simulink model "SEWSYS_Combined"  (Simulink 6.0)
settings: Solver=FixedStepDiscrete  SolverMode=SingleTasking  StartTime=0  StopTime=Q  FixedStep=1  RelTol=1e-3
values from neighbouring files (symbols this model uses):
  andpt = 1/3    (= 0.333333333333)    [constants_trafik.m]
  andt = 0.1    [constants_trafik.m]
  baseflow = str2num(get(HH, 'String'))    [inputs.m]
  CSO_limit = in_CSO_limit    [Prep.m]
  delayinit = [zeros(1,nr_ex_H2O)]    [constants_trafik.m]
  fast = 0.7    [constants_trafik.m]
  fkmday = in_fkmday    [areas.m]
  init_init = 4*3600    (= 14400)    [areas.m]
  init_time = 5    [areas.m]
  nhv = in_nhv/100    [areas.m]
  nr_ex_H2O = totnr-1    (= 20)    [Prep.m]
  numberOfPersons = in_numberOfPersons    [Prep.m]
  othera = in_otherarea    [areas.m]
  othermax = drydepmax*othera    [constants_trafik.m]
  redu = 0.8    [areas.m]
  roada = in_roads    [areas.m]
  roadaccmax = dryper*24*sph*fast*(p_tyrewear+p_roadwear+p_exhaust+p_breakwear+p_drydep+p_corrZn+p_oildischarge+p_catalyst)    [constants_trafik.m]
  roadkm = 67e9    (= 67000000000)    [constants_trafik.m]
  roadrunpart = 1    [constants_trafik.m]
  roadwear = 130000    [constants_trafik.m]
  roadZna = in_part_roadZna/100*roada    [areas.m]
  roofa = in_roofs    [areas.m]
  RoofCua = in_part_roofCua/100*roofa/cos(15*pi/180)    [areas.m]
  roofmax = (Znroofmax*RoofZna+Curoofmax*RoofCua)*roofrunpart+drydepmax*roofa    [constants_trafik.m]
  roofrunpart = 0.7    [constants_trafik.m]
  RoofZna = in_part_roofZna/100*roofa/cos(15*pi/180)    [areas.m]
  sec_per_ts = in_sec_per_ts    [Prep.m]
  sph = 3600/sec_per_ts    [Prep.m]
  tota = in_tota    [areas.m]
  totnr = 21    [Prep.m]
  tyrewear = 9000    [constants_trafik.m]
  wetdep = [sum(s_wetdep(:,i))]*tota*trans1    [polldistr_gr.m]
  yearly_rain = 1    [Callback_simulate.m]    (also in SEWSYS_fig.m)
undefined symbols (not defined in the file or in its folder): BDT, BODofVS, brakep, catalystp, CSO_choice, Curoofp, DiscIntNeverNeededParam, Drainage, drydep, exhp, Faeces, Industry, K, oilp, ProcSS_bio, ProcSS_chem, ProcSS_presed, ProcSS_sand, ProcSS_screen, roadp, sani, spBiooxidBod, spBiored, spCcontent, spChemFe, spChemicalPart, spCODBOD, spDenSS, spHeavym, spHjust, spN2ONpurEmitted, spNemitted, spNitrif, spNpur, spOcontent, spPBound, spPout, spPout1, spVSofSS, SSred_bio, SSred_chem, SSred_presed, SSred_sand, SSred_screen, SStoWater, stormw, tyrep, Urine, VSofSS_sand, VSofSS_screen, Znroofp
(part 1 of 2)
settings Model: LastModifiedBy=v94ahlst  ExtModeTrigMode=oneshot  ExtModeArmWhenConnect=off
settings DataIOCC: LimitDataPoints=off  SignalLoggingName=sigsOut
settings OptimizationCC: BlockReduction=off  BooleanDataType=off
settings DebuggingCC: SolverPrmCheckMsg=none
settings HardwareCC: TargetUnknown=on
settings GRTTargetCC: ModelReferenceCompliant=off  MatFileLogging=off

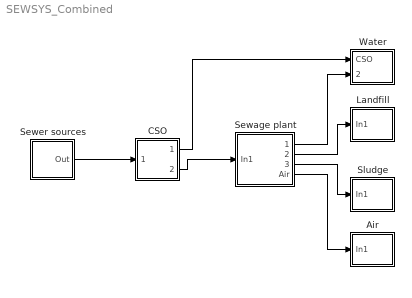
== system SEWSYS_Combined ==
  Air : Subsystem
  CSO : Subsystem
  Landfill : Subsystem
  Sewage plant : Subsystem
  Sewer sources : Subsystem
  Sludge : Subsystem
  Water : Subsystem
  wires:
  Sewage plant/2(Landfill) -> Landfill/1(In1)
  Sewage plant/3(Sludge) -> Sludge/1(In1)
  Sewage plant/1(" Wastewater") -> Water/2(WWTP)
  Sewage plant/4(Air) -> Air/1(In1)
  Sewer sources/1(Out) -> CSO/1(In1)
  CSO/1(Out1) -> Water/1(CSO)
  CSO/2("Out2 ") -> Sewage plant/1(In1)

== system SEWSYS_Combined/Air ==
  In1 : Inport  Port=1  LatchInput=off
  To Workspace : ToWorkspace  VariableName=outAir  SampleTime=-1  SaveFormat=Array
  wires:
  In1/1 -> To Workspace/1

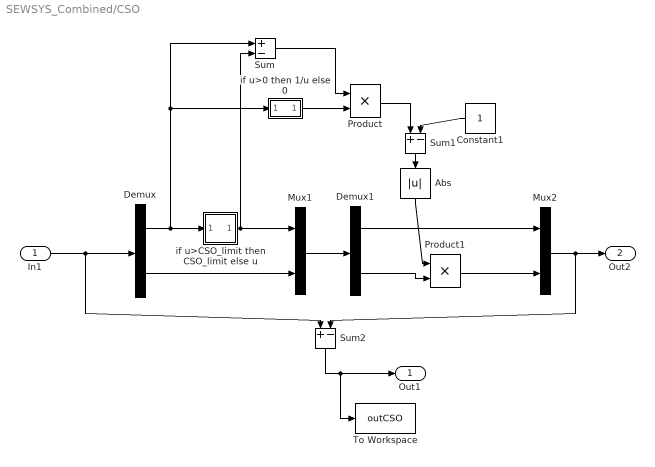
== system SEWSYS_Combined/CSO ==
  In1 : Inport  Port=1  LatchInput=off
  Abs : Abs  Orientation=down  SaturateOnIntegerOverflow=on
  Constant1 : Constant  Orientation=left
  Demux : Demux  Outputs=[1 -1]
  Demux1 : Demux  Outputs=[1 -1]
  Mux1 : Mux  Inputs=2
  Mux2 : Mux  Inputs=2
  Product : Product  SaturateOnIntegerOverflow=on  InputSameDT=on
  Product1 : Product  SaturateOnIntegerOverflow=on  InputSameDT=on
  Sum : Sum  Inputs=+-  SaturateOnIntegerOverflow=on  InputSameDT=on
  Sum1 : Sum  Orientation=down  Inputs=+-  SaturateOnIntegerOverflow=on  InputSameDT=on
  Sum2 : Sum  Orientation=down  Inputs=+-  SaturateOnIntegerOverflow=on  InputSameDT=on
  To Workspace : ToWorkspace  VariableName=outCSO  SampleTime=-1  SaveFormat=Array
  if u>0 then 1/u else 0 : Subsystem
      mask Display: disp('1/u')
  if u>CSO_limit then CSO_limit else u : Subsystem
      mask Display: disp('CSO')
  Out1 : Outport
  "Out2 " : Outport  Port=2
  wires:
  Demux/2 -> Mux1/2
  Mux1/1 -> Demux1/1
  Demux1/1 -> Mux2/1
  Demux1/2 -> Product1/2
  Product1/1 -> Mux2/2
  if u>CSO_limit then CSO_limit else u/1(out_1) -> Sum/2, Mux1/1
  Constant1/1 -> Sum1/2
  Demux/1 -> if u>CSO_limit then CSO_limit else u/1(in_1), Sum/1, if u>0 then 1/u else 0/1(in_1)
  Sum1/1 -> Abs/1
  if u>0 then 1/u else 0/1(out_1) -> Product/2
  Sum2/1 -> Out1/1, To Workspace/1
  In1/1 -> Demux/1, Sum2/1
  Mux2/1 -> "Out2 "/1, Sum2/2
  Product/1 -> Sum1/1
  Abs/1 -> Product1/1
  Sum/1 -> Product/1

== system SEWSYS_Combined/Landfill ==
  In1 : Inport  Port=1  LatchInput=off
  To Workspace : ToWorkspace  VariableName=outLandfill  SampleTime=-1  SaveFormat=Array
  wires:
  In1/1 -> To Workspace/1

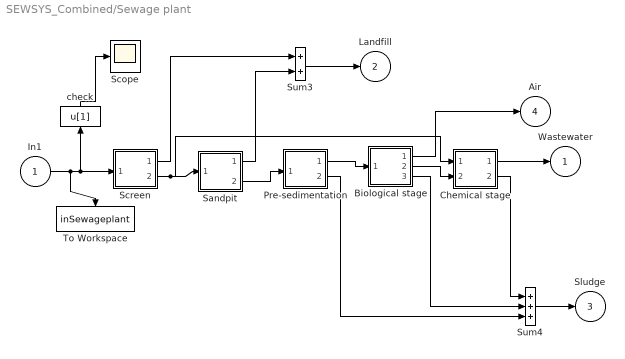
== system SEWSYS_Combined/Sewage plant ==
  In1 : Inport  Port=1  LatchInput=off
  Biological stage : Subsystem
  Chemical stage : Subsystem
  Pre-sedimentation : Subsystem
  Sandpit : Subsystem
  Scope : Scope
  Screen : Subsystem
  Sum3 : Sum  SaturateOnIntegerOverflow=on  InputSameDT=on
  Sum4 : Sum  Inputs=+++  SaturateOnIntegerOverflow=on  InputSameDT=on
  To Workspace : ToWorkspace  VariableName=inSewageplant  SampleTime=-1  SaveFormat=Array
      settings: Orientation=down
  check : Fcn  Orientation=up  Expr=u[1]
  " Wastewater" : Outport
  Landfill : Outport  Port=2
  Sludge : Outport  Port=3
  Air : Outport  Port=4
  wires:
  In1/1 -> To Workspace/1, Screen/1(In1), check/1
  Sum3/1 -> Landfill/1
  Screen/2(Out2) -> Chemical stage/1(In1), Sandpit/1(In1)
  Sum4/1 -> Sludge/1
  Screen/1(Out1) -> Sum3/1
  Sandpit/2(Out2) -> Pre-sedimentation/1(In1)
  Chemical stage/1(Out1) -> " Wastewater"/1
  Biological stage/1(Airemission) -> Air/1
  Biological stage/2(Wastewater) -> Chemical stage/2(In2)
  Pre-sedimentation/1(Out1) -> Biological stage/1(in_1)
  Sandpit/1(Out1) -> Sum3/2
  Biological stage/3(Biosludge) -> Sum4/2
  Chemical stage/2(Out2) -> Sum4/1
  Pre-sedimentation/2(Out2) -> Sum4/3
  check/1 -> Scope/1

== system SEWSYS_Combined/Sewer sources ==
  Apply time-series : Subsystem
  Drainage : Subsystem
  "Sani choice " : Gain  Gain=sani  SaturateOnIntegerOverflow=on
  Sanitary wastewater : Subsystem
  Storm Choice : Gain  Gain=stormw  SaturateOnIntegerOverflow=on
  Storm water : Subsystem
  Sum : Sum  SaturateOnIntegerOverflow=on  InputSameDT=on
  Sum1 : Sum  SaturateOnIntegerOverflow=on  InputSameDT=on
  Sum2 : Sum  SaturateOnIntegerOverflow=on  InputSameDT=on
  To Workspace5 : ToWorkspace  VariableName=storm  SampleTime=-1  SaveFormat=Array
      settings: Orientation=down
  To Workspace6 : ToWorkspace  VariableName=sewer  SampleTime=-1  SaveFormat=Array
      settings: Orientation=down
  Out : Outport
  wires:
  Sanitary wastewater/2(Out2) -> Sum/2
  Storm water/1(Storm Water [m3/s] pollutants [g/s]) -> Storm Choice/1
  Storm Choice/1 -> Sum1/2, To Workspace5/1
  Sum1/1 -> Out/1
  "Sani choice "/1 -> Sum1/1, To Workspace6/1
  Sanitary wastewater/1(Out1) -> Sum/1
  Sum/1 -> Apply time-series/1(In1)
  Sum2/1 -> "Sani choice "/1
  Drainage/1(Out) -> Sum2/2
  Apply time-series/1(Out1) -> Sum2/1

== system SEWSYS_Combined/Sludge ==
  In1 : Inport  Port=1  LatchInput=off
  To Workspace : ToWorkspace  VariableName=outSludge  SampleTime=-1  SaveFormat=Array
  wires:
  In1/1 -> To Workspace/1

== system SEWSYS_Combined/Water ==
  CSO : Inport  Port=1  LatchInput=off
  WWTP : Inport  Port=2  LatchInput=off
  Sum : Sum  SaturateOnIntegerOverflow=on  InputSameDT=on
  To Workspace : ToWorkspace  VariableName=outRecipient  SampleTime=-1  SaveFormat=Array
  To Workspace1 : ToWorkspace  VariableName=out_WWTP_Recipient  SampleTime=-1  SaveFormat=Array
  wires:
  CSO/1 -> Sum/1
  Sum/1 -> To Workspace/1
  WWTP/1 -> Sum/2, To Workspace1/1

== system SEWSYS_Combined/CSO/if u>0 then 1/u else 0 ==
  note: if u<=0, 0, else 1/u, end
  in_1 : Inport  Orientation=left  Port=1  LatchInput=off
  Constant : Constant  Orientation=left  Value=0
  Constant1 : Constant  Orientation=left
  Switch : Switch  Orientation=left  SaturateOnIntegerOverflow=on  InputSameDT=on
  Switch1 : Switch  Orientation=left  SaturateOnIntegerOverflow=on  InputSameDT=on
  inv. : Fcn  Orientation=left  Expr=1/u
  neg : Gain  Orientation=left  Gain=-1  SaturateOnIntegerOverflow=on
  neg1 : Gain  Orientation=left  Gain=-1  SaturateOnIntegerOverflow=on
  out_1 : Outport  Orientation=left  InitialOutput=0
  wires:
  Constant/1 -> Switch/1
  neg/1 -> Switch/2
  Switch/1 -> out_1/1
  inv./1 -> Switch/3
  Switch1/1 -> inv./1
  neg1/1 -> Switch1/2
  Constant1/1 -> Switch1/1
  in_1/1 -> neg/1, neg1/1, Switch1/3

== system SEWSYS_Combined/CSO/if u>CSO_limit then CSO_limit else u ==
  note: if u>=CSO_limit, CSO_limit
      | , else u, end
  note: if CSO_choice>=1, CSO, else u, end
  in_1 : Inport  Port=1  LatchInput=off
  CSO : Switch  Threshold=CSO_limit  SaturateOnIntegerOverflow=on  InputSameDT=on
  Constant : Constant  Value=CSO_limit
  Constant1 : Constant  Value=CSO_choice
  choice : Switch  Threshold=1  SaturateOnIntegerOverflow=on  InputSameDT=on
  inv. : Fcn  Expr=u
  out_1 : Outport  InitialOutput=0
  wires:
  Constant1/1 -> choice/2
  Constant/1 -> CSO/1
  inv./1 -> CSO/3
  CSO/1 -> choice/1
  in_1/1 -> CSO/2, inv./1, choice/3
  choice/1 -> out_1/1

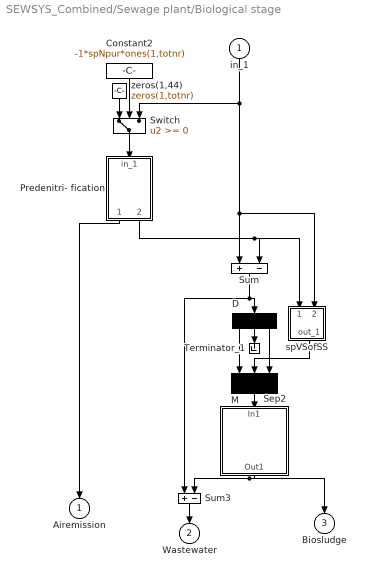
== system SEWSYS_Combined/Sewage plant/Biological stage ==
  in_1 : Inport  Orientation=down  Port=1  LatchInput=off
  Constant2 : Constant  Orientation=down  Value=-1*spNpur*ones(1,totnr)
      mask Display: disp('spNpur')
  D : Demux  Orientation=down  Outputs=NewVSofSS
  M : Mux  Orientation=down  Inputs=NewVSofSS
  Predenitri- fication : Subsystem  Orientation=down
      mask Display: plot([0,5,5,0,0],[0,0,10,10,0],[0,0.8],[6,6],[1.3,2.3],[6,6],[2.8,3.8],[6,6],[4.3,5],[6,6],[5,8,8,5,5.5,5.5,5],[1,1,9,9,9.2,8.8,9])
  Sep2 : Subsystem  Orientation=down
  Sum : Sum  Orientation=down  Inputs=+-  SaturateOnIntegerOverflow=on  InputSameDT=on
  Sum3 : Sum  Orientation=down  Inputs=+-  SaturateOnIntegerOverflow=on  InputSameDT=on
  "Switch " : Switch  Orientation=down  SaturateOnIntegerOverflow=on  InputSameDT=on
  Terminator_1 : Terminator
      settings: Orientation=down
  spVSofSS : Subsystem  Orientation=down
  "zeros(1,44) " : Constant  Orientation=down  Value=zeros(1,totnr)
      mask Display: disp('0')
  Airemission : Outport  Orientation=down  InitialOutput=0
  Wastewater : Outport  Orientation=down  Port=2  InitialOutput=0
  Biosludge : Outport  Orientation=down  Port=3  InitialOutput=0
  wires:
  D/1 -> M/1
  "zeros(1,44) "/1 -> "Switch "/1
  Constant2/1 -> "Switch "/2
  Sum/1 -> D/1, Sum3/1
  D/2 -> Terminator_1/1
  Predenitri- fication/1(ToAir) -> Airemission/1
  M/1 -> Sep2/1(In1)
  Sum3/1 -> Wastewater/1
  D/3 -> M/3
  Sep2/1(Out1) -> Sum3/2, Biosludge/1
  in_1/1 -> spVSofSS/2(in_2), Sum/1, "Switch "/3
  "Switch "/1 -> Predenitri- fication/1(in_1)
  Predenitri- fication/2(Reduction of wastewater) -> spVSofSS/1(in_1), Sum/2
  spVSofSS/1(out_1) -> M/2

== system SEWSYS_Combined/Sewage plant/Chemical stage ==
  In1 : Inport  Port=1  LatchInput=off
  In2 : Inport  Port=2  LatchInput=off
  "BOD,  COD" : MATLABFcn  MATLABFcn=[zeros(size(1:7)) , u(8)*(1-0.97), u(9)*(1-0.93),zeros(size(1:12))]
  BOD=0 COD=0 : MATLABFcn  MATLABFcn=[u(1:7) ; 0; 0; u(10:21)]
  Separation : Subsystem
  Sum : Sum  Inputs=++-  SaturateOnIntegerOverflow=on  InputSameDT=on
  Out1 : Outport
  Out2 : Outport  Port=2
  wires:
  Sum/1 -> Out1/1
  BOD=0 COD=0/1 -> Sum/2
  In1/1 -> "BOD,  COD"/1
  "BOD,  COD"/1 -> Sum/1
  Separation/1(Out1) -> Sum/3, Out2/1
  In2/1 -> BOD=0 COD=0/1, Separation/1(In1)

== system SEWSYS_Combined/Sewage plant/Pre-sedimentation ==
  In1 : Inport  Port=1  LatchInput=off
  Chemical : Subsystem
  Demux : Demux  Outputs=NewVSofSS
  Mux : Mux  Inputs=NewVSofSS
  Separation : Subsystem
  Sum : Sum  Inputs=+-  SaturateOnIntegerOverflow=on  InputSameDT=on
  Sum1 : Sum  SaturateOnIntegerOverflow=on  InputSameDT=on
  Terminator_1 : Terminator
  spVSofSS : Subsystem
  Out1 : Outport
  Out2 : Outport  Port=2
  wires:
  Sum1/1 -> Demux/1
  Demux/2 -> Terminator_1/1
  Demux/1 -> Mux/1
  Demux/3 -> Mux/3
  In1/1 -> Chemical/1(in_1), Sum1/2, spVSofSS/2(in_2), Separation/2(In2)
  Mux/1 -> Sum/1, Separation/1(In1)
  Separation/1(Out1) -> Out2/1, Sum/2
  Sum/1 -> Out1/1
  Chemical/1(out_1) -> spVSofSS/1(in_1), Sum1/1
  spVSofSS/1(out_1) -> Mux/2

== system SEWSYS_Combined/Sewage plant/Sandpit ==
  In1 : Inport  Port=1  LatchInput=off
  Separation : Subsystem
  Sum : Sum  Inputs=-+  SaturateOnIntegerOverflow=on  InputSameDT=on
  Out1 : Outport
  Out2 : Outport  Port=2
  wires:
  In1/1 -> Separation/1(In1), Sum/2
  Separation/1(Out1) -> Out1/1, Sum/1
  Sum/1 -> Out2/1

== system SEWSYS_Combined/Sewage plant/Screen ==
  In1 : Inport  Port=1  LatchInput=off
  Separation : Subsystem
  Sum : Sum  Inputs=-+  SaturateOnIntegerOverflow=on  InputSameDT=on
  Out1 : Outport
  Out2 : Outport  Port=2
  wires:
  In1/1 -> Separation/1(In1), Sum/2
  Separation/1(Out1) -> Out1/1, Sum/1
  Sum/1 -> Out2/1

== system SEWSYS_Combined/Sewer sources/Apply time-series ==
  In1 : Inport  Port=1  LatchInput=off
  Demux : Demux  Outputs=2
  Mux1 : Mux  Inputs=[1,nr_ex_H2O]
  Product1 : Product  SaturateOnIntegerOverflow=on  InputSameDT=on
  Product2 : Product  SaturateOnIntegerOverflow=on  InputSameDT=on
  SewVar (factors) : FromWorkspace  Orientation=down  VariableName=[T,U1]  SampleTime=1
  Out1 : Outport
  wires:
  In1/1 -> Demux/1
  Mux1/1 -> Out1/1
  Product2/1 -> Mux1/2  "nr_ex_H2O]"
  Demux/1 -> Product1/2
  Demux/2 -> Product2/2
  Product1/1 -> Mux1/1  "[1"
  SewVar (factors)/1 -> Product1/1, Product2/1

== system SEWSYS_Combined/Sewer sources/Drainage ==
  Drainage : Constant  Value=Drainage
  Out : Outport
  wires:
  Drainage/1 -> Out/1

== system SEWSYS_Combined/Sewer sources/Sanitary wastewater ==
  Household : Subsystem
  Industry : Subsystem
  Out1 : Outport
  Out2 : Outport  Port=2
  wires:
  Industry/1(Out) -> Out2/1
  Household/1(Out) -> Out1/1

== system SEWSYS_Combined/Sewer sources/Storm water ==
  Add Baseflow : Subsystem
  Add pollutants in rain : Subsystem
  From Workspace : FromWorkspace  VariableName=[T,U2]  SampleTime=1
  Make per second : Subsystem
  "Rain -> Stormwater" : Subsystem
  Runoff : Subsystem
  To Workspace6 : ToWorkspace  VariableName=storm1  SampleTime=-1  SaveFormat=Array
      settings: Orientation=down
  Storm Water [m3/s] pollutants [g/s] : Outport
  wires:
  From Workspace/1 -> Add pollutants in rain/1(rain [mm])
  Add pollutants in rain/1(rain [mm] pollutants [ug/m2]) -> "Rain -> Stormwater"/1("rain[mm] pollutants [ug/m2] ")
  Make per second/1(Out1) -> Runoff/1("In1 ")
  "Rain -> Stormwater"/1("SW[m3] pollutants [g] ") -> Make per second/1(In1), To Workspace6/1
  Runoff/1(Out1) -> Add Baseflow/1("In1 ")
  Add Baseflow/1(Out1) -> Storm Water [m3/s] pollutants [g/s]/1

== system SEWSYS_Combined/Sewage plant/Biological stage/Predenitri- fication ==
  note: Ändrat så också SS bryts ned
      |  vid oxidering av kol till CO2
  in_1 : Inport  Orientation=down  Port=1  LatchInput=off
  Aeration and degradation of PP. gradation of SS  PP*(BioSep(1)+BioSep(2)) SS=u(6)*0,75*(Biograd-Bioass), : MATLABFcn  Orientation=down  MATLABFcn=[ zeros(6,1); -u(8)*spBiored*(1-spBiooxidBod)/(spCcontent*2*16/12-spOcontent); zeros(14,1)]
  Change from  NH4 to NO3 : MATLABFcn  Orientation=down  MATLABFcn=[zeros(3,1); u(4)*spNemitted*spNitrif; -u(4)*spNemitted*spNitrif ;zeros(16,1)]
  "Consumption of  BOD, COD, Ctot, Cch.. " : MATLABFcn  Orientation=down  MATLABFcn="u(8)*spBiooxidBod*spBiored*(12)/(2*16)/spCcontent.*[zeros(6,1); spDenSS;  spCcontent*(2*16)/12; spCcontent*(2*16)/12; spCcontent; zeros(11,1)]"
  "Emissions of CO2, through assimilation of VS, and PP to air u(8)*BioassBOD*(12+2*16)/(2*16), PP*BioSep(1)" : MATLABFcn  Orientation=down  MATLABFcn=[zeros(9,1); u(8)*spBiooxidBod*spBiored*12/(2*16); zeros(11,1)]
  N-org to NH4 through oxid to CO2 : Subsystem  Orientation=down
  NH3 emissions from  aeration to nitrification  and degration of BOD. : Subsystem  Orientation=down
  Nitrification/ denitrification : Subsystem  Orientation=down
  Sum : Sum  Orientation=down  Inputs=+++  SaturateOnIntegerOverflow=on  InputSameDT=on
  Sum1 : Sum  Orientation=down  Inputs=+-++++  SaturateOnIntegerOverflow=on  InputSameDT=on
  Sum2 : Sum  Orientation=down  Inputs=+-  SaturateOnIntegerOverflow=on  InputSameDT=on
  ToAir : Outport  Orientation=down  InitialOutput=0
  Reduction of wastewater : Outport  Orientation=down  Port=2  InitialOutput=0
  wires:
  Sum1/1 -> Reduction of wastewater/1
  in_1/1 -> NH3 emissions from  aeration to nitrification  and degration of BOD./1(in_1), Sum2/1, Nitrification/ denitrification/1(in_1)
  N-org to NH4 through oxid to CO2/1(Out1) -> Sum1/2
  Sum2/1 -> "Emissions of CO2, through assimilation of VS, and PP to air u(8)*BioassBOD*(12+2*16)/(2*16), PP*BioSep(1)"/1, NH3 emissions from  aeration to nitrification  and degration of BOD./2(in_2), Change from  NH4 to NO3/1, "Consumption of  BOD, COD, Ctot, Cch.. "/1, Aeration and degradation of PP. gradation of SS  PP*(BioSep(1)+BioSep(2)) SS=u(6)*0,75*(Biograd-Bioass),/1, N-org to NH4 through oxid to CO2/2(In2)
  Aeration and degradation of PP. gradation of SS  PP*(BioSep(1)+BioSep(2)) SS=u(6)*0,75*(Biograd-Bioass),/1 -> Sum1/3
  Sum/1 -> ToAir/1
  NH3 emissions from  aeration to nitrification  and degration of BOD./1(out_1) -> Sum/3, Sum1/1
  "Consumption of  BOD, COD, Ctot, Cch.. "/1 -> Sum1/4
  "Emissions of CO2, through assimilation of VS, and PP to air u(8)*BioassBOD*(12+2*16)/(2*16), PP*BioSep(1)"/1 -> Sum/2, N-org to NH4 through oxid to CO2/1(In1)
  Nitrification/ denitrification/1(ToAir) -> Sum/1
  Change from  NH4 to NO3/1 -> Sum1/5
  Nitrification/ denitrification/2(Reduction of wastewater) -> Sum1/6, Sum2/2

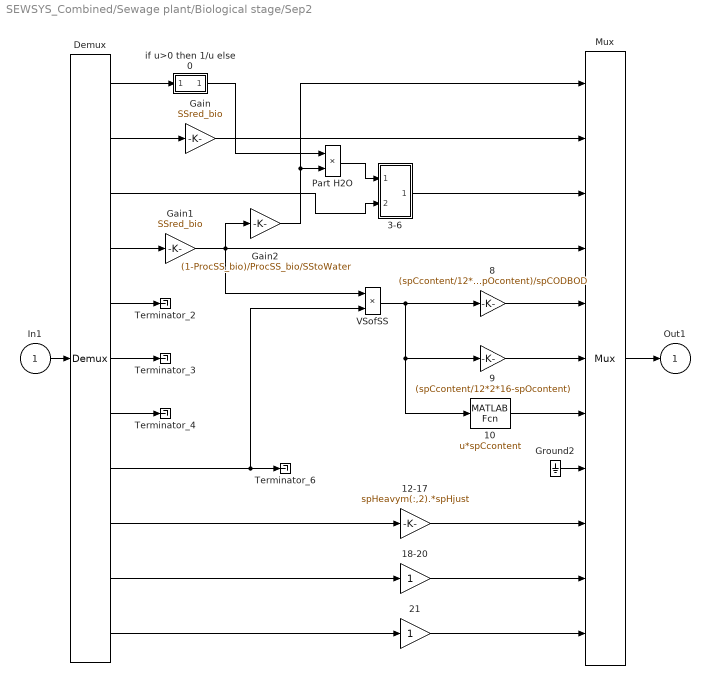
== system SEWSYS_Combined/Sewage plant/Biological stage/Sep2 ==
  In1 : Inport  Port=1  LatchInput=off
  10 : MATLABFcn  MATLABFcn=u*spCcontent
  12-17 : Gain  Gain=spHeavym(:,2).*spHjust  SaturateOnIntegerOverflow=on
  18-20 : Gain  SaturateOnIntegerOverflow=on
  21 : Gain  SaturateOnIntegerOverflow=on
  3-6 : Subsystem
      mask Display: disp('N')
  8 : Gain  Gain=(spCcontent/12*2*16-spOcontent)/spCODBOD  SaturateOnIntegerOverflow=on
  9 : Gain  Gain=(spCcontent/12*2*16-spOcontent)  SaturateOnIntegerOverflow=on
  Demux : Demux  Outputs=Separation
  Gain : Gain  Gain=SSred_bio  SaturateOnIntegerOverflow=on
  Gain1 : Gain  Gain=SSred_bio  SaturateOnIntegerOverflow=on
  Gain2 : Gain  Gain=(1-ProcSS_bio)/ProcSS_bio/SStoWater  SaturateOnIntegerOverflow=on
  Ground2 : Ground
  Mux : Mux  Inputs=Separation
  Part H2O : Product  SaturateOnIntegerOverflow=on  InputSameDT=on
  Terminator_{2..4,6} (4 alike) : Terminator
  VSofSS : Product  SaturateOnIntegerOverflow=on  InputSameDT=on
  if u>0 then 1/u else 0 : Subsystem
      mask Display: disp('1/u')
  Out1 : Outport
  wires:
  Demux/4 -> Gain1/1
  Demux/7 -> Terminator_4/1
  Demux/8 -> VSofSS/2, Terminator_6/1
  Gain1/1 -> VSofSS/1, Mux/4, Gain2/1
  Demux/6 -> Terminator_3/1
  Demux/5 -> Terminator_2/1
  if u>0 then 1/u else 0/1(out_1) -> Part H2O/1
  Demux/3 -> 3-6/2("in_2 ")
  Part H2O/1 -> 3-6/1(in_1)
  In1/1 -> Demux/1
  Demux/2 -> Gain/1
  Demux/1 -> if u>0 then 1/u else 0/1(in_1)
  VSofSS/1 -> 8/1, 9/1, 10/1
  Gain2/1 -> Mux/1, Part H2O/2
  Demux/9 -> 12-17/1
  10/1 -> Mux/7
  Ground2/1 -> Mux/8
  9/1 -> Mux/6
  8/1 -> Mux/5
  3-6/1(out_1) -> Mux/3
  Mux/1 -> Out1/1
  Gain/1 -> Mux/2
  12-17/1 -> Mux/9
  Demux/10 -> 18-20/1
  18-20/1 -> Mux/10
  Demux/11 -> 21/1
  21/1 -> Mux/11

== system SEWSYS_Combined/Sewage plant/Biological stage/spVSofSS ==
  in_1 : Inport  Orientation=down  Port=1  LatchInput=off
  in_2 : Inport  Orientation=down  Port=2  LatchInput=off
  17 : Product  Orientation=down  SaturateOnIntegerOverflow=on  InputSameDT=on
  18 : Product  Orientation=down  SaturateOnIntegerOverflow=on  InputSameDT=on
  Sum7 : Sum  Orientation=down  SaturateOnIntegerOverflow=on  InputSameDT=on
  Sum8 : Sum  Orientation=down  SaturateOnIntegerOverflow=on  InputSameDT=on
  if u>0 then 1/u else 0 : Subsystem  Orientation=down
      mask Display: disp('1/u')
  spBioSS : Fcn  Orientation=down  Expr=-u[7]
  spSS : Fcn  Orientation=down  Expr=u[7]
  spVSofSS : Fcn  Orientation=down  Expr=u[11]
  out_1 : Outport  Orientation=down  InitialOutput=0
  wires:
  in_1/1 -> spBioSS/1
  in_2/1 -> spSS/1, spVSofSS/1
  Sum7/1 -> 17/1
  17/1 -> out_1/1
  spVSofSS/1 -> 18/1
  spSS/1 -> Sum8/2, 18/2
  Sum8/1 -> if u>0 then 1/u else 0/1(in_1)
  if u>0 then 1/u else 0/1(out_1) -> 17/2
  spBioSS/1 -> Sum8/1, Sum7/1
  18/1 -> Sum7/2

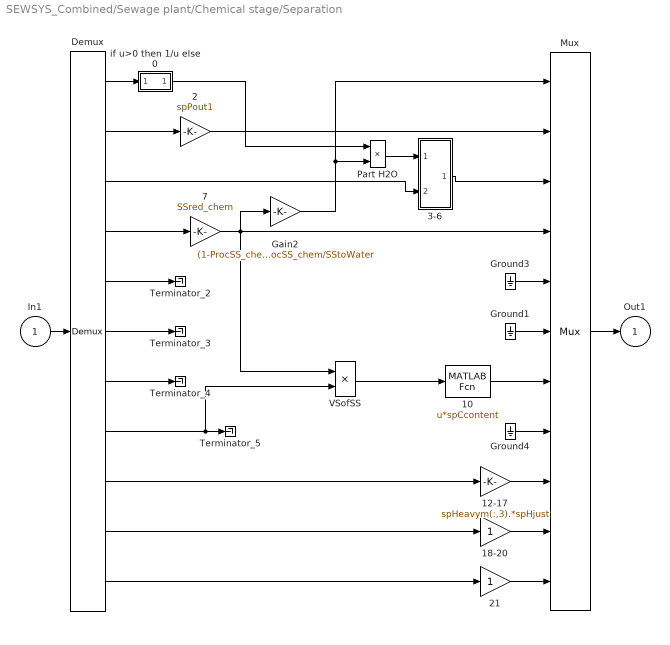
== system SEWSYS_Combined/Sewage plant/Chemical stage/Separation ==
  In1 : Inport  Port=1  LatchInput=off
  10 : MATLABFcn  MATLABFcn=u*spCcontent
  12-17 : Gain  Gain=spHeavym(:,3).*spHjust  SaturateOnIntegerOverflow=on
  18-20 : Gain  SaturateOnIntegerOverflow=on
  2 : Gain  Gain=spPout1  SaturateOnIntegerOverflow=on
  21 : Gain  SaturateOnIntegerOverflow=on
  3-6 : Subsystem
      mask Display: disp('N')
  7 : Gain  Gain=SSred_chem  SaturateOnIntegerOverflow=on
  Demux : Demux  Outputs=Separation
  Gain2 : Gain  Gain=(1-ProcSS_chem)/ProcSS_chem/SStoWater  SaturateOnIntegerOverflow=on
  Ground1 : Ground
  Ground3 : Ground
  Ground4 : Ground
  Mux : Mux  Inputs=Separation
  Part H2O : Product  SaturateOnIntegerOverflow=on  InputSameDT=on
  Terminator_{2..5} (4 alike) : Terminator
  VSofSS : Product  SaturateOnIntegerOverflow=on  InputSameDT=on
  if u>0 then 1/u else 0 : Subsystem
      mask Display: disp('1/u')
  Out1 : Outport
  wires:
  Demux/1 -> if u>0 then 1/u else 0/1(in_1)
  Demux/2 -> 2/1
  In1/1 -> Demux/1
  Demux/4 -> 7/1
  Part H2O/1 -> 3-6/1(in_1)
  Demux/3 -> 3-6/2("in_2 ")
  if u>0 then 1/u else 0/1(out_1) -> Part H2O/1
  Demux/5 -> Terminator_2/1
  Demux/6 -> Terminator_3/1
  Demux/7 -> Terminator_4/1
  Demux/8 -> Terminator_5/1, VSofSS/2
  7/1 -> VSofSS/1, Mux/4, Gain2/1
  Gain2/1 -> Mux/1, Part H2O/2
  2/1 -> Mux/2
  Mux/1 -> Out1/1
  3-6/1(out_1) -> Mux/3
  Ground3/1 -> Mux/5
  Ground1/1 -> Mux/6
  Ground4/1 -> Mux/8
  10/1 -> Mux/7
  VSofSS/1 -> 10/1
  Demux/9 -> 12-17/1
  12-17/1 -> Mux/9
  Demux/10 -> 18-20/1
  18-20/1 -> Mux/10
  Demux/11 -> 21/1
  21/1 -> Mux/11

== system SEWSYS_Combined/Sewage plant/Pre-sedimentation/Chemical ==
  in_1 : Inport  Port=1  LatchInput=off
  Amount of chemical : Fcn  Orientation=up  Expr=u(2)*(1.1-spPout)/0.56*(55.55/31)/spChemFe
  Chemical : MATLABFcn  MATLABFcn=spChemicalPart.*u/1000  OutputDimensions=totnr
  Chemsludge : MATLABFcn  MATLABFcn=[zeros(6,1); u(2)*spPBound*(30.97+55.85+16.0*4)/30.97; zeros(14,1)]
  Demux : Demux  Outputs=[1,nr_ex_H2O]
  H20 g/s - m3/s : Fcn  Expr=u(1)/1000000
  More Info : Subsystem
      mask Display: disp('Info')
  Mux : Mux  Inputs=[1,nr_ex_H2O]
  Sum : Sum  SaturateOnIntegerOverflow=on  InputSameDT=on
  To Workspace6 : ToWorkspace  VariableName=chem  SampleTime=-1  SaveFormat=Array
  out_1 : Outport  InitialOutput=0
  wires:
  Sum/1 -> out_1/1
  Chemsludge/1 -> Sum/2
  Amount of chemical/1 -> Chemical/1
  Chemical/1 -> Demux/1
  Demux/1 -> H20 g/s - m3/s/1
  H20 g/s - m3/s/1 -> Mux/1
  Demux/2 -> Mux/2
  Mux/1 -> Sum/1, To Workspace6/1
  in_1/1 -> Chemsludge/1, Amount of chemical/1

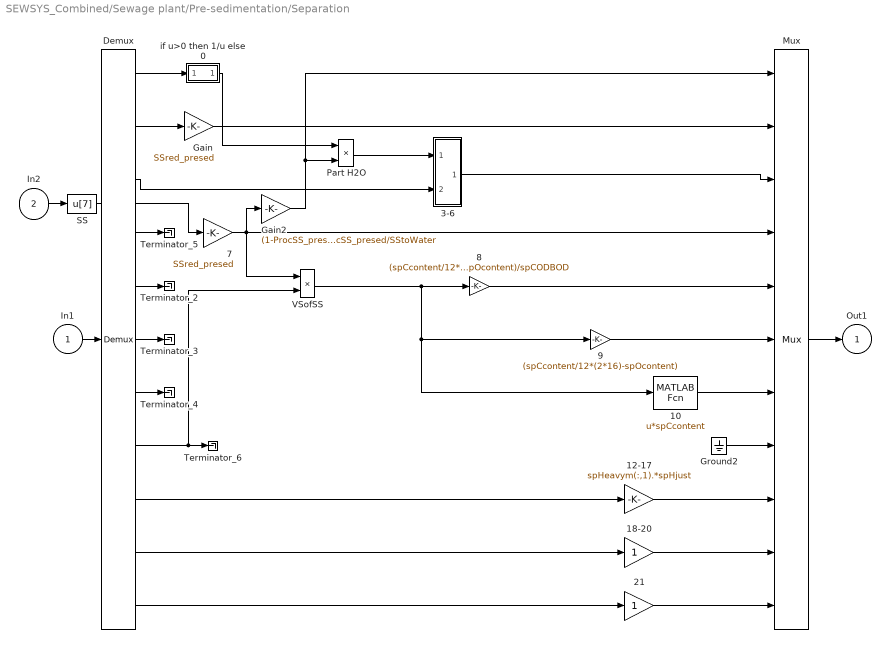
== system SEWSYS_Combined/Sewage plant/Pre-sedimentation/Separation ==
  In1 : Inport  Port=1  LatchInput=off
  In2 : Inport  Port=2  LatchInput=off
  10 : MATLABFcn  MATLABFcn=u*spCcontent
  12-17 : Gain  Gain=spHeavym(:,1).*spHjust  SaturateOnIntegerOverflow=on
  18-20 : Gain  SaturateOnIntegerOverflow=on
  21 : Gain  SaturateOnIntegerOverflow=on
  3-6 : Subsystem
      mask Display: disp('N')
  7 : Gain  Gain=SSred_presed  SaturateOnIntegerOverflow=on
  8 : Gain  Gain=(spCcontent/12*(2*16)-spOcontent)/spCODBOD  SaturateOnIntegerOverflow=on
  9 : Gain  Gain=(spCcontent/12*(2*16)-spOcontent)  SaturateOnIntegerOverflow=on
  Demux : Demux  Outputs=Separation
  Gain : Gain  Gain=SSred_presed  SaturateOnIntegerOverflow=on
  Gain2 : Gain  Gain=(1-ProcSS_presed)/ProcSS_presed/SStoWater  SaturateOnIntegerOverflow=on
  Ground2 : Ground
  Mux : Mux  Inputs=Separation
  Part H2O : Product  SaturateOnIntegerOverflow=on  InputSameDT=on
  "SS " : Fcn  Expr=u[7]
  Terminator_{2..6} (5 alike) : Terminator
  VSofSS : Product  SaturateOnIntegerOverflow=on  InputSameDT=on
  if u>0 then 1/u else 0 : Subsystem
      mask Display: disp('1/u')
  Out1 : Outport
  wires:
  Demux/1 -> if u>0 then 1/u else 0/1(in_1)
  Demux/2 -> Gain/1
  Gain/1 -> Mux/2
  Mux/1 -> Out1/1
  In1/1 -> Demux/1
  Part H2O/1 -> 3-6/1(in_1)
  Demux/3 -> 3-6/2("in_2 ")
  if u>0 then 1/u else 0/1(out_1) -> Part H2O/1
  Demux/5 -> Terminator_2/1
  8/1 -> Mux/5
  Demux/6 -> Terminator_3/1
  9/1 -> Mux/6
  Demux/4 -> Terminator_5/1
  "SS "/1 -> 7/1
  Ground2/1 -> Mux/8
  Demux/7 -> Terminator_4/1
  10/1 -> Mux/7
  12-17/1 -> Mux/9
  Demux/9 -> 12-17/1
  In2/1 -> "SS "/1
  7/1 -> Mux/4, Gain2/1, VSofSS/1
  Demux/8 -> Terminator_6/1, VSofSS/2
  VSofSS/1 -> 8/1, 9/1, 10/1
  Gain2/1 -> Mux/1, Part H2O/2
  3-6/1(out_1) -> Mux/3
  18-20/1 -> Mux/10
  Demux/10 -> 18-20/1
  Demux/11 -> 21/1
  21/1 -> Mux/11

== system SEWSYS_Combined/Sewage plant/Pre-sedimentation/spVSofSS ==
  in_1 : Inport  Port=1  LatchInput=off
  in_2 : Inport  Port=2  LatchInput=off
  17 : Product  SaturateOnIntegerOverflow=on  InputSameDT=on
  Sum7 : Sum  SaturateOnIntegerOverflow=on  InputSameDT=on
  if u>0 then 1/u else 0 : Subsystem
      mask Display: disp('1/u')
  spChemSS : Fcn  Expr=u[7]
  spSS : Fcn  Expr=u[7]
  spVS : Gain  Gain=spVSofSS  SaturateOnIntegerOverflow=on
  out_1 : Outport  InitialOutput=0
  wires:
  in_1/1 -> spChemSS/1
  in_2/1 -> spSS/1
  spVS/1 -> 17/2
  17/1 -> out_1/1
  spChemSS/1 -> Sum7/1
  if u>0 then 1/u else 0/1(out_1) -> 17/1
  spSS/1 -> spVS/1, Sum7/2
  Sum7/1 -> if u>0 then 1/u else 0/1(in_1)

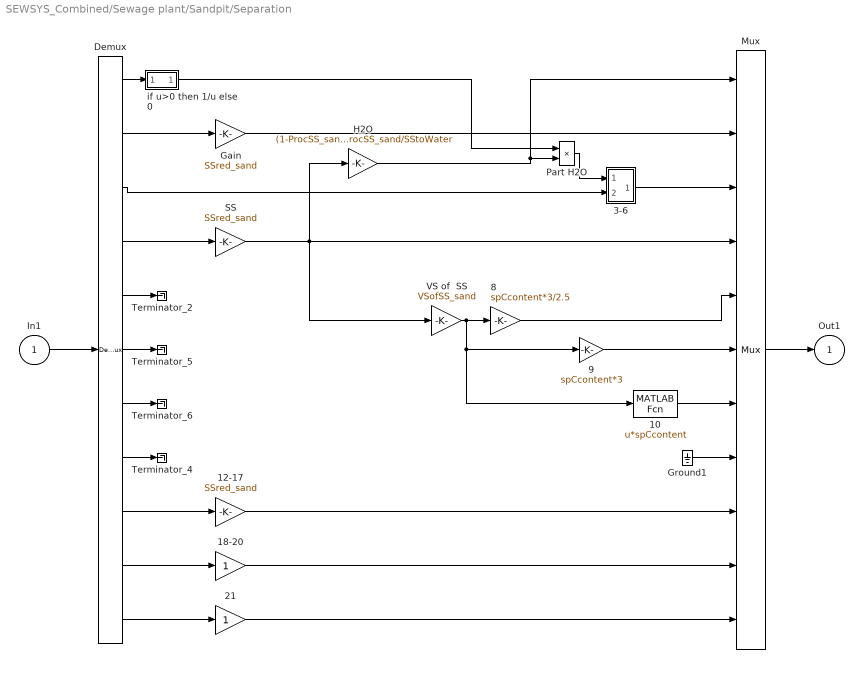
== system SEWSYS_Combined/Sewage plant/Sandpit/Separation ==
  In1 : Inport  Port=1  LatchInput=off
  10 : MATLABFcn  MATLABFcn=u*spCcontent
  12-17 : Gain  Gain=SSred_sand  SaturateOnIntegerOverflow=on
  18-20 : Gain  SaturateOnIntegerOverflow=on
  21 : Gain  SaturateOnIntegerOverflow=on
  3-6 : Subsystem
      mask Display: disp('N')
  8 : Gain  Gain=spCcontent*3/2.5  SaturateOnIntegerOverflow=on
  9 : Gain  Gain=spCcontent*3  SaturateOnIntegerOverflow=on
  Demux : Demux  Outputs=Separation
  Gain : Gain  Gain=SSred_sand  SaturateOnIntegerOverflow=on
  Ground1 : Ground
  H2O : Gain  Gain=(1-ProcSS_sand)/ProcSS_sand/SStoWater  SaturateOnIntegerOverflow=on
  Mux : Mux  Inputs=Separation
  Part H2O : Product  SaturateOnIntegerOverflow=on  InputSameDT=on
  SS : Gain  Gain=SSred_sand  SaturateOnIntegerOverflow=on
  Terminator_{2,4..6} (4 alike) : Terminator
  VS of  SS : Gain  Gain=VSofSS_sand  SaturateOnIntegerOverflow=on
  if u>0 then 1/u else 0 : Subsystem
      mask Display: disp('1/u')
  Out1 : Outport
  wires:
  10/1 -> Mux/7
  Demux/8 -> Terminator_4/1
  9/1 -> Mux/6
  8/1 -> Mux/5
  3-6/1(out_1) -> Mux/3
  Demux/4 -> SS/1
  In1/1 -> Demux/1
  Mux/1 -> Out1/1
  Gain/1 -> Mux/2
  Demux/2 -> Gain/1
  Demux/1 -> if u>0 then 1/u else 0/1(in_1)
  VS of  SS/1 -> 8/1, 9/1, 10/1
  Part H2O/1 -> 3-6/1(in_1)
  if u>0 then 1/u else 0/1(out_1) -> Part H2O/1
  SS/1 -> Mux/4, VS of  SS/1, H2O/1
  Demux/3 -> 3-6/2("in_2 ")
  H2O/1 -> Mux/1, Part H2O/2
  Demux/9 -> 12-17/1
  12-17/1 -> Mux/9
  Demux/7 -> Terminator_6/1
  Demux/6 -> Terminator_5/1
  Demux/5 -> Terminator_2/1
  Ground1/1 -> Mux/8
  Demux/10 -> 18-20/1
  18-20/1 -> Mux/10
  Demux/11 -> 21/1
  21/1 -> Mux/11

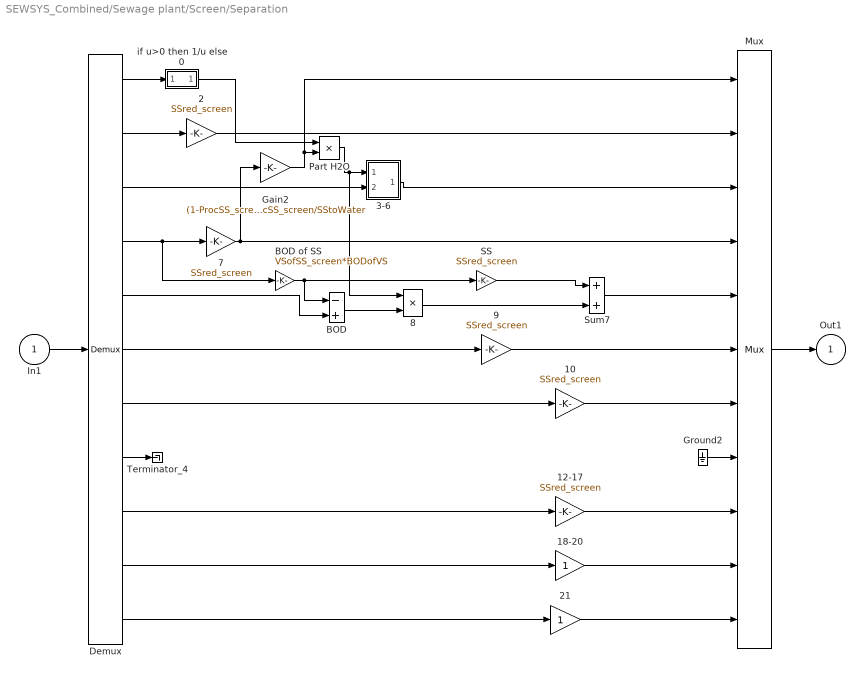
== system SEWSYS_Combined/Sewage plant/Screen/Separation ==
  In1 : Inport  Port=1  LatchInput=off
  {2,7,9..10} (4 alike) : Gain  Gain=SSred_screen  SaturateOnIntegerOverflow=on
  12-17 : Gain  Gain=SSred_screen  SaturateOnIntegerOverflow=on
  18-20 : Gain  SaturateOnIntegerOverflow=on
  21 : Gain  SaturateOnIntegerOverflow=on
  3-6 : Subsystem
      mask Display: disp('N')
  8 : Product  SaturateOnIntegerOverflow=on  InputSameDT=on
  BOD : Sum  Inputs=-+  SaturateOnIntegerOverflow=on  InputSameDT=on
  BOD of SS : Gain  Gain=VSofSS_screen*BODofVS  SaturateOnIntegerOverflow=on
  Demux : Demux  Outputs=Separation
  Gain2 : Gain  Gain=(1-ProcSS_screen)/ProcSS_screen/SStoWater  SaturateOnIntegerOverflow=on
  Ground2 : Ground
  Mux : Mux  Inputs=Separation
  Part H2O : Product  SaturateOnIntegerOverflow=on  InputSameDT=on
  SS : Gain  Gain=SSred_screen  SaturateOnIntegerOverflow=on
  Sum7 : Sum  SaturateOnIntegerOverflow=on  InputSameDT=on
  Terminator_4 : Terminator
  if u>0 then 1/u else 0 : Subsystem
      mask Display: disp('1/u')
  Out1 : Outport
  wires:
  In1/1 -> Demux/1
  Mux/1 -> Out1/1
  Demux/2 -> 2/1
  Demux/1 -> if u>0 then 1/u else 0/1(in_1)
  Sum7/1 -> Mux/5
  Demux/6 -> 9/1
  9/1 -> Mux/6
  Ground2/1 -> Mux/8
  Demux/7 -> 10/1
  10/1 -> Mux/7
  Demux/8 -> Terminator_4/1
  2/1 -> Mux/2
  SS/1 -> Sum7/1
  Demux/5 -> BOD/2
  7/1 -> Mux/4, Gain2/1
  3-6/1(out_1) -> Mux/3
  if u>0 then 1/u else 0/1(out_1) -> Part H2O/1
  Demux/3 -> 3-6/2("in_2 ")
  Demux/4 -> 7/1, BOD of SS/1
  BOD/1 -> 8/2
  Part H2O/1 -> 3-6/1(in_1), 8/1
  BOD of SS/1 -> SS/1, BOD/1
  8/1 -> Sum7/2
  Gain2/1 -> Part H2O/2, Mux/1
  Demux/9 -> 12-17/1
  12-17/1 -> Mux/9
  Demux/10 -> 18-20/1
  18-20/1 -> Mux/10
  Demux/11 -> 21/1
  21/1 -> Mux/11

== system SEWSYS_Combined/Sewer sources/Sanitary wastewater/Household ==
  Greywater : Subsystem
  Product : Product  SaturateOnIntegerOverflow=on  InputSameDT=on
  Sum : Sum  SaturateOnIntegerOverflow=on  InputSameDT=on
  Toilet : Subsystem
  numberOfPersons : Constant  Value=numberOfPersons
  Out : Outport
  wires:
  Toilet/1(Out) -> Sum/1
  Greywater/1(Out) -> Sum/2
  Sum/1 -> Product/1
  Product/1 -> Out/1
  numberOfPersons/1 -> Product/2

== system SEWSYS_Combined/Sewer sources/Sanitary wastewater/Industry ==
  "Industry " : Constant  Value=Industry
  To Workspace6 : ToWorkspace  VariableName=s_industry  SampleTime=-1  SaveFormat=Array
  Out : Outport
  wires:
  "Industry "/1 -> Out/1, To Workspace6/1

== system SEWSYS_Combined/Sewer sources/Storm water/Add Baseflow ==
  "In1 " : Inport  Port=1  LatchInput=off
  Baseflow : Constant  Value=baseflow
  Demux : Demux  Outputs=[1 -1]
  Mux1 : Mux  Inputs=2
  Sum : Sum  SaturateOnIntegerOverflow=on  InputSameDT=on
  Out1 : Outport
  wires:
  Demux/2 -> Mux1/2
  Sum/1 -> Mux1/1
  Mux1/1 -> Out1/1
  "In1 "/1 -> Demux/1
  Baseflow/1 -> Sum/1
  Demux/1 -> Sum/2

== system SEWSYS_Combined/Sewer sources/Storm water/Add pollutants in rain ==
  rain [mm] : Inport  Port=1  LatchInput=off
  Initial loss : Subsystem
  reduction factor : Gain  Gain=redu  SaturateOnIntegerOverflow=on
  wet deposition : Subsystem
  rain [mm] pollutants [ug/m2] : Outport
  wires:
  rain [mm]/1 -> Initial loss/1(rain [mm])
  reduction factor/1 -> wet deposition/1(rain [mm])
  wet deposition/1(rain [mm] pollutants [ug/m2]) -> rain [mm] pollutants [ug/m2]/1
  Initial loss/1(rain  [mm]) -> reduction factor/1

== system SEWSYS_Combined/Sewer sources/Storm water/Make per second ==
  In1 : Inport  Port=1  LatchInput=off
  Demux : Demux  Outputs=[1 -1]
  Mux1 : Mux  Inputs=2
  g - g/s : Gain  Gain=1/sec_per_ts  SaturateOnIntegerOverflow=on
  m3 - m3/s : Gain  Gain=1/sec_per_ts  SaturateOnIntegerOverflow=on
  Out1 : Outport
  wires:
  In1/1 -> Demux/1
  Mux1/1 -> Out1/1
  Demux/1 -> m3 - m3/s/1
  m3 - m3/s/1 -> Mux1/1
  Demux/2 -> g - g/s/1
  g - g/s/1 -> Mux1/2

== system SEWSYS_Combined/Sewer sources/Storm water/Rain -> Stormwater ==
  "rain[mm] pollutants [ug/m2] " : Inport  Port=1  LatchInput=off
  Sum : Sum  Inputs=+++  SaturateOnIntegerOverflow=on  InputSameDT=on
  other surfaces : Subsystem
  road surfaces : Subsystem
  roofs : Subsystem
  "SW[m3] pollutants [g] " : Outport
  wires:
  road surfaces/1(rain[m3] pollutants [g]) -> Sum/1
  "rain[mm] pollutants [ug/m2] "/1 -> road surfaces/1(rain [mm] pollutants [ug/m2]1), other surfaces/1(rain[mm] pollutants [ug/m2]), roofs/1(rain [mm]  pollutants[ug/m2])
  Sum/1 -> "SW[m3] pollutants [g] "/1
  roofs/1(rain[m3] pollutants [g]) -> Sum/2
  other surfaces/1(rain[m3] pollutants [g]) -> Sum/3

== system SEWSYS_Combined/Sewer sources/Storm water/Runoff ==
  "In1 " : Inport  Port=1  LatchInput=off
  Demux : Demux  Outputs=[1 -1]
  Mux1 : Mux  Inputs=2
  Subsystem1 : Subsystem
  Out1 : Outport
  wires:
  "In1 "/1 -> Demux/1
  Mux1/1 -> Out1/1
  Demux/1 -> Subsystem1/1(In1)
  Subsystem1/1(Out1) -> Mux1/1
  Demux/2 -> Mux1/2

== system SEWSYS_Combined/Sewage plant/Biological stage/Predenitri- fication/N-org to NH4 through oxid to CO2 ==
  In1 : Inport  Orientation=down  Port=1  LatchInput=off
  In2 : Inport  Orientation=down  Port=2  LatchInput=off
  C-tot : Fcn  Orientation=down  Expr=u(10)
  Ctot degr. : Fcn  Orientation=down  Expr=u(10)
  N-org : Fcn  Orientation=down  Expr=u(3)-u(4)-u(5)
  N-org degraded  to NH4 : Product  Orientation=down  SaturateOnIntegerOverflow=on  InputSameDT=on
  NH4 increased : MATLABFcn  Orientation=down  MATLABFcn=[zeros(3,1); u ; zeros(17,1)]  OutputDimensions=totnr
  Part of C-tot degraded : Product  Orientation=down  SaturateOnIntegerOverflow=on  InputSameDT=on
  if u>0 then 1/u else 0 : Subsystem  Orientation=down
      mask Display: disp('1/u')
  Out1 : Outport  Orientation=down  InitialOutput=0
  wires:
  N-org/1 -> N-org degraded  to NH4/2
  Part of C-tot degraded/1 -> N-org degraded  to NH4/1
  Ctot degr./1 -> Part of C-tot degraded/1
  In1/1 -> Ctot degr./1
  C-tot/1 -> if u>0 then 1/u else 0/1(in_1)
  if u>0 then 1/u else 0/1(out_1) -> Part of C-tot degraded/2
  In2/1 -> C-tot/1, N-org/1
  N-org degraded  to NH4/1 -> NH4 increased/1
  NH4 increased/1 -> Out1/1

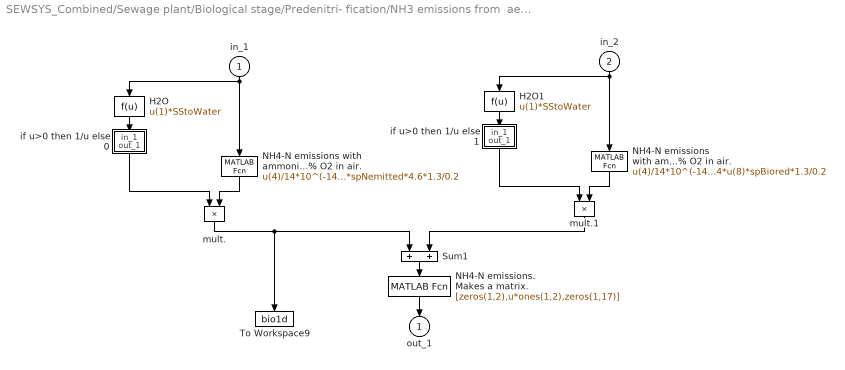
== system SEWSYS_Combined/Sewage plant/Biological stage/Predenitri- fication/NH3 emissions from  aeration to nitrification  and degration of BOD. ==
  in_1 : Inport  Orientation=down  Port=1  LatchInput=off
  in_2 : Inport  Orientation=down  Port=2  LatchInput=off
  H2O : Fcn  Orientation=down  Expr=u(1)*SStoWater
  H2O1 : Fcn  Orientation=down  Expr=u(1)*SStoWater
  "NH4-N emissions  with ammonia  in equilibrium with air in the baisin Aeration with 1.3 kg O2/kg BOD  degr.and 20% O2 in air. " : MATLABFcn  Orientation=down  MATLABFcn=u(4)/14*10^(-1477.7/288+1.6937)*0.0831*288/(1+10^(-7.7)/10^(-0.09018-2729.92/288))*696.4*u(8)*spBiored*1.3/0.2  OutputDimensions=1
  NH4-N emissions with ammonia  in equilibrium with air in the baisin Aeration with 4.6*1.3 kg O2/kg N  emitted and 20% O2 in air. : MATLABFcn  Orientation=down  MATLABFcn=u(4)/14*10^(-1477.7/288+1.6937)*0.0831*288/(1+10^(-7.7)/10^(-0.09018-2729.92/288))*696.4*u(3)*spNemitted*4.6*1.3/0.2  OutputDimensions=1
  NH4-N emissions. Makes a matrix. : MATLABFcn  Orientation=down  MATLABFcn=[zeros(1,2),u*ones(1,2),zeros(1,17)]  OutputDimensions=totnr
  Sum1 : Sum  Orientation=down  SaturateOnIntegerOverflow=on  InputSameDT=on
  To Workspace9 : ToWorkspace  VariableName=bio1d  SampleTime=-1  SaveFormat=Array
      settings: Orientation=down
  if u>0 then 1/u else 0 : Subsystem  Orientation=down
      mask Display: disp('1/u')
  if u>0 then 1/u else 1 : Subsystem  Orientation=down
      mask Display: disp('1/u')
  mult. : Product  Orientation=down  SaturateOnIntegerOverflow=on  InputSameDT=on
  mult.1 : Product  Orientation=down  SaturateOnIntegerOverflow=on  InputSameDT=on
  out_1 : Outport  Orientation=down  InitialOutput=0
  wires:
  mult./1 -> To Workspace9/1, Sum1/1
  mult.1/1 -> Sum1/2
  Sum1/1 -> NH4-N emissions. Makes a matrix./1
  NH4-N emissions. Makes a matrix./1 -> out_1/1
  in_1/1 -> NH4-N emissions with ammonia  in equilibrium with air in the baisin Aeration with 4.6*1.3 kg O2/kg N  emitted and 20% O2 in air./1, H2O/1
  NH4-N emissions with ammonia  in equilibrium with air in the baisin Aeration with 4.6*1.3 kg O2/kg N  emitted and 20% O2 in air./1 -> mult./2
  if u>0 then 1/u else 0/1(out_1) -> mult./1
  H2O/1 -> if u>0 then 1/u else 0/1(in_1)
  H2O1/1 -> if u>0 then 1/u else 1/1(in_1)
  if u>0 then 1/u else 1/1(out_1) -> mult.1/1
  "NH4-N emissions  with ammonia  in equilibrium with air in the baisin Aeration with 1.3 kg O2/kg BOD  degr.and 20% O2 in air. "/1 -> mult.1/2
  in_2/1 -> H2O1/1, "NH4-N emissions  with ammonia  in equilibrium with air in the baisin Aeration with 1.3 kg O2/kg BOD  degr.and 20% O2 in air. "/1

== system SEWSYS_Combined/Sewage plant/Biological stage/Predenitri- fication/Nitrification/ denitrification ==
  note: CO2 Utsläpp borttagen
  note: Är allt kol som förbrukas
      | bundet till VS?
  in_1 : Inport  Orientation=down  Port=1  LatchInput=off
  BOD and COD consumed : MATLABFcn  Orientation=down  MATLABFcn="u/14*5/4*(2*16)*[zeros(7,1); 1;  1; zeros(12,1)]"  OutputDimensions=totnr
  C-consumed : MATLABFcn  Orientation=down  MATLABFcn=[zeros(9,1); u*5/4*12/14; zeros(11,1)]  OutputDimensions=totnr
  N-efficiency : Fcn  Orientation=down  Expr=u(3)*spNemitted
  N-org to NH4 : Subsystem  Orientation=down
  N-reduction due to N2O and N2 emitted : MATLABFcn  Orientation=down  MATLABFcn="[zeros(2,1); u(3)*(spN2ONpurEmitted+spNemitted);u(4)*(spN2ONpurEmitted+spNemitted);  zeros(17,1)]"
  N2-N-emitted : MATLABFcn  Orientation=down  MATLABFcn=[zeros(2,1); u; zeros(18,1)]  OutputDimensions=totnr
  N2O-N-emitted : MATLABFcn  Orientation=down  MATLABFcn=[zeros(2,1); u(3)*spN2ONpurEmitted; zeros(2,1); u(3)*spN2ONpurEmitted; zeros(15,1)]
  Sum1 : Sum  Orientation=down  SaturateOnIntegerOverflow=on  InputSameDT=on
  Sum2 : Sum  Orientation=down  Inputs=+-++  SaturateOnIntegerOverflow=on  InputSameDT=on
  VS/TS-consumed : MATLABFcn  Orientation=down  MATLABFcn=u(10)/spCcontent*[zeros(6,1); spDenSS ;zeros(2,1); spCcontent; zeros(11,1)]
  ToAir : Outport  Orientation=down  InitialOutput=0
  Reduction of wastewater : Outport  Orientation=down  Port=2  InitialOutput=0
  wires:
  N-reduction due to N2O and N2 emitted/1 -> Sum2/4
  in_1/1 -> N2O-N-emitted/1, N-efficiency/1, N-reduction due to N2O and N2 emitted/1, N-org to NH4/2(In2)
  N2-N-emitted/1 -> Sum1/2
  N2O-N-emitted/1 -> Sum1/1
  Sum1/1 -> ToAir/1
  N-efficiency/1 -> N2-N-emitted/1, BOD and COD consumed/1, C-consumed/1
  Sum2/1 -> Reduction of wastewater/1
  VS/TS-consumed/1 -> Sum2/1
  BOD and COD consumed/1 -> Sum2/3
  C-consumed/1 -> VS/TS-consumed/1, N-org to NH4/1(In1)
  N-org to NH4/1(Out1) -> Sum2/2

== system SEWSYS_Combined/Sewage plant/Biological stage/Sep2/3-6 ==
  in_1 : Inport  Orientation=down  Port=1  LatchInput=off
  "in_2 " : Inport  Orientation=down  Port=2  LatchInput=off
  Ground1 : Ground  Orientation=down
  Mux : Mux  Orientation=down
  N-tot : MATLABFcn  Orientation=down  MATLABFcn=(u(1)-u(2)-u(3))*SSred_bio  OutputDimensions=1
  NH4 : Product  Orientation=down  SaturateOnIntegerOverflow=on  InputSameDT=on
  "NH4 " : Fcn  Orientation=down  Expr=u(2)
  NH5 : Product  Orientation=down  SaturateOnIntegerOverflow=on  InputSameDT=on
  NO3 : Fcn  Orientation=down  Expr=u(3)
  Sum : Sum  Orientation=down  Inputs=+++  SaturateOnIntegerOverflow=on  InputSameDT=on
  out_1 : Outport  Orientation=down  InitialOutput=0
  wires:
  Ground1/1 -> Mux/4
  NH5/1 -> Mux/3, Sum/3
  "in_2 "/1 -> N-tot/1, "NH4 "/1, NO3/1
  NO3/1 -> NH5/2
  "NH4 "/1 -> NH4/2
  Sum/1 -> Mux/1
  N-tot/1 -> Sum/1
  Mux/1 -> out_1/1
  in_1/1 -> NH4/1, NH5/1
  NH4/1 -> Sum/2, Mux/2

== system SEWSYS_Combined/Sewage plant/Biological stage/Sep2/if u>0 then 1/u else 0 ==
  note: if u<=0, 0, else 1/u, end
  in_1 : Inport  Orientation=left  Port=1  LatchInput=off
  Constant : Constant  Orientation=left  Value=0
  Constant1 : Constant  Orientation=left
  Switch : Switch  Orientation=left  SaturateOnIntegerOverflow=on  InputSameDT=on
  Switch1 : Switch  Orientation=left  SaturateOnIntegerOverflow=on  InputSameDT=on
  inv. : Fcn  Orientation=left  Expr=1/u
  neg : Gain  Orientation=left  Gain=-1  SaturateOnIntegerOverflow=on
  neg1 : Gain  Orientation=left  Gain=-1  SaturateOnIntegerOverflow=on
  out_1 : Outport  Orientation=left  InitialOutput=0
  wires:
  Switch/1 -> out_1/1
  neg/1 -> Switch/2
  Constant/1 -> Switch/1
  inv./1 -> Switch/3
  Switch1/1 -> inv./1
  neg1/1 -> Switch1/2
  Constant1/1 -> Switch1/1
  in_1/1 -> neg/1, neg1/1, Switch1/3

== system SEWSYS_Combined/Sewage plant/Biological stage/spVSofSS/if u>0 then 1/u else 0 ==
  note: if u<=0, 0, else 1/u, end
  in_1 : Inport  Orientation=left  Port=1  LatchInput=off
  Constant : Constant  Orientation=left  Value=0
  Constant1 : Constant  Orientation=left
  Switch : Switch  Orientation=left  SaturateOnIntegerOverflow=on  InputSameDT=on
  Switch1 : Switch  Orientation=left  SaturateOnIntegerOverflow=on  InputSameDT=on
  inv. : Fcn  Orientation=left  Expr=1/u
  neg : Gain  Orientation=left  Gain=-1  SaturateOnIntegerOverflow=on
  neg1 : Gain  Orientation=left  Gain=-1  SaturateOnIntegerOverflow=on
  out_1 : Outport  Orientation=left  InitialOutput=0
  wires:
  Switch/1 -> out_1/1
  inv./1 -> Switch/3
  neg/1 -> Switch/2
  Constant/1 -> Switch/1
  Switch1/1 -> inv./1
  neg1/1 -> Switch1/2
  Constant1/1 -> Switch1/1
  in_1/1 -> neg/1, neg1/1, Switch1/3

== system SEWSYS_Combined/Sewage plant/Chemical stage/Separation/3-6 ==
  in_1 : Inport  Orientation=down  Port=1  LatchInput=off
  "in_2 " : Inport  Orientation=down  Port=2  LatchInput=off
  Ground1 : Ground  Orientation=down
  Mux : Mux  Orientation=down
  N-tot : MATLABFcn  Orientation=down  MATLABFcn=(u(1)-u(2)-u(3))*SSred_chem  OutputDimensions=1
  NH4 : Product  Orientation=down  SaturateOnIntegerOverflow=on  InputSameDT=on
  "NH4 " : Fcn  Orientation=down  Expr=u(2)
  NH5 : Product  Orientation=down  SaturateOnIntegerOverflow=on  InputSameDT=on
  NO3 : Fcn  Orientation=down  Expr=u(3)
  Sum : Sum  Orientation=down  Inputs=+++  SaturateOnIntegerOverflow=on  InputSameDT=on
  out_1 : Outport  Orientation=down  InitialOutput=0
  wires:
  NH4/1 -> Mux/2, Sum/2
  in_1/1 -> NH5/1, NH4/1
  Mux/1 -> out_1/1
  N-tot/1 -> Sum/1
  Sum/1 -> Mux/1
  "NH4 "/1 -> NH4/2
  NO3/1 -> NH5/2
  "in_2 "/1 -> NO3/1, "NH4 "/1, N-tot/1
  NH5/1 -> Sum/3, Mux/3
  Ground1/1 -> Mux/4

== system SEWSYS_Combined/Sewage plant/Chemical stage/Separation/if u>0 then 1/u else 0 ==
  note: if u<=0, 0, else 1/u, end
  in_1 : Inport  Orientation=left  Port=1  LatchInput=off
  Constant : Constant  Orientation=left  Value=0
  Constant1 : Constant  Orientation=left
  Switch : Switch  Orientation=left  SaturateOnIntegerOverflow=on  InputSameDT=on
  Switch1 : Switch  Orientation=left  SaturateOnIntegerOverflow=on  InputSameDT=on
  inv. : Fcn  Orientation=left  Expr=1/u
  neg : Gain  Orientation=left  Gain=-1  SaturateOnIntegerOverflow=on
  neg1 : Gain  Orientation=left  Gain=-1  SaturateOnIntegerOverflow=on
  out_1 : Outport  Orientation=left  InitialOutput=0
  wires:
  Constant/1 -> Switch/1
  neg/1 -> Switch/2
  Switch/1 -> out_1/1
  inv./1 -> Switch/3
  Switch1/1 -> inv./1
  neg1/1 -> Switch1/2
  Constant1/1 -> Switch1/1
  in_1/1 -> neg/1, neg1/1, Switch1/3

== system SEWSYS_Combined/Sewage plant/Pre-sedimentation/Chemical/More Info ==
  note: Checked 940314
  note: Amount of chemical is calculated and sent to workspace in spChemicalInput
      | It is calculated from a special input per cubic meter wastewater.
      | The chemical (PIX-C) is modulated as  water with some heavymetal.

== system SEWSYS_Combined/Sewage plant/Pre-sedimentation/Separation/3-6 ==
  in_1 : Inport  Orientation=down  Port=1  LatchInput=off
  "in_2 " : Inport  Orientation=down  Port=2  LatchInput=off
  Ground1 : Ground  Orientation=down
  Mux : Mux  Orientation=down
  N-tot : MATLABFcn  Orientation=down  MATLABFcn=(u(1)-u(2)-u(3))*SSred_presed  OutputDimensions=1
  NH4 : Product  Orientation=down  SaturateOnIntegerOverflow=on  InputSameDT=on
  "NH4 " : Fcn  Orientation=down  Expr=u(2)
  NH5 : Product  Orientation=down  SaturateOnIntegerOverflow=on  InputSameDT=on
  NO3 : Fcn  Orientation=down  Expr=u(3)
  Sum : Sum  Orientation=down  Inputs=+++  SaturateOnIntegerOverflow=on  InputSameDT=on
  out_1 : Outport  Orientation=down  InitialOutput=0
  wires:
  NH4/1 -> Mux/2, Sum/2
  in_1/1 -> NH5/1, NH4/1
  Mux/1 -> out_1/1
  N-tot/1 -> Sum/1
  Sum/1 -> Mux/1
  "NH4 "/1 -> NH4/2
  NO3/1 -> NH5/2
  "in_2 "/1 -> NO3/1, "NH4 "/1, N-tot/1
  NH5/1 -> Sum/3, Mux/3
  Ground1/1 -> Mux/4

== system SEWSYS_Combined/Sewage plant/Pre-sedimentation/Separation/if u>0 then 1/u else 0 ==
  note: if u<=0, 0, else 1/u, end
  in_1 : Inport  Orientation=left  Port=1  LatchInput=off
  Constant : Constant  Orientation=left  Value=0
  Constant1 : Constant  Orientation=left
  Switch : Switch  Orientation=left  SaturateOnIntegerOverflow=on  InputSameDT=on
  Switch1 : Switch  Orientation=left  SaturateOnIntegerOverflow=on  InputSameDT=on
  inv. : Fcn  Orientation=left  Expr=1/u
  neg : Gain  Orientation=left  Gain=-1  SaturateOnIntegerOverflow=on
  neg1 : Gain  Orientation=left  Gain=-1  SaturateOnIntegerOverflow=on
  out_1 : Outport  Orientation=left  InitialOutput=0
  wires:
  Constant/1 -> Switch/1
  neg/1 -> Switch/2
  Switch/1 -> out_1/1
  inv./1 -> Switch/3
  Switch1/1 -> inv./1
  neg1/1 -> Switch1/2
  Constant1/1 -> Switch1/1
  in_1/1 -> neg/1, neg1/1, Switch1/3

== system SEWSYS_Combined/Sewage plant/Pre-sedimentation/spVSofSS/if u>0 then 1/u else 0 ==
  note: if u<=0, 0, else 1/u, end
  in_1 : Inport  Orientation=left  Port=1  LatchInput=off
  Constant : Constant  Orientation=left  Value=0
  Constant1 : Constant  Orientation=left
  Switch : Switch  Orientation=left  SaturateOnIntegerOverflow=on  InputSameDT=on
  Switch1 : Switch  Orientation=left  SaturateOnIntegerOverflow=on  InputSameDT=on
  To Workspace6 : ToWorkspace  VariableName=otest1  SampleTime=-1  SaveFormat=Array
  inv. : Fcn  Orientation=left  Expr=1/u
  neg : Gain  Orientation=left  Gain=-1  SaturateOnIntegerOverflow=on
  neg1 : Gain  Orientation=left  Gain=-1  SaturateOnIntegerOverflow=on
  out_1 : Outport  Orientation=left  InitialOutput=0
  wires:
  inv./1 -> Switch/3
  Constant/1 -> Switch/1
  neg/1 -> Switch/2, To Workspace6/1
  Switch1/1 -> inv./1
  Switch/1 -> out_1/1
  neg1/1 -> Switch1/2
  Constant1/1 -> Switch1/1
  in_1/1 -> neg/1, neg1/1, Switch1/3

== system SEWSYS_Combined/Sewage plant/Sandpit/Separation/3-6 ==
  in_1 : Inport  Orientation=down  Port=1  LatchInput=off
  "in_2 " : Inport  Orientation=down  Port=2  LatchInput=off
  Ground2 : Ground  Orientation=down
  Mux : Mux  Orientation=down
  N-tot : MATLABFcn  Orientation=down  MATLABFcn=(u(1)-u(2)-u(3))*SSred_sand  OutputDimensions=1
  NH4 : Product  Orientation=down  SaturateOnIntegerOverflow=on  InputSameDT=on
  "NH4 " : Fcn  Orientation=down  Expr=u(2)
  NH5 : Product  Orientation=down  SaturateOnIntegerOverflow=on  InputSameDT=on
  NO3 : Fcn  Orientation=down  Expr=u(3)
  Sum : Sum  Orientation=down  Inputs=+++  SaturateOnIntegerOverflow=on  InputSameDT=on
  out_1 : Outport  Orientation=down  InitialOutput=0
  wires:
  Ground2/1 -> Mux/4
  NH5/1 -> Mux/3, Sum/3
  "in_2 "/1 -> N-tot/1, "NH4 "/1, NO3/1
  NO3/1 -> NH5/2
  "NH4 "/1 -> NH4/2
  Sum/1 -> Mux/1
  N-tot/1 -> Sum/1
  Mux/1 -> out_1/1
  in_1/1 -> NH4/1, NH5/1
  NH4/1 -> Sum/2, Mux/2

== system SEWSYS_Combined/Sewage plant/Sandpit/Separation/if u>0 then 1/u else 0 ==
  note: if u<=0, 0, else 1/u, end
  in_1 : Inport  Orientation=left  Port=1  LatchInput=off
  Constant : Constant  Orientation=left  Value=0
  Constant1 : Constant  Orientation=left
  Switch : Switch  Orientation=left  SaturateOnIntegerOverflow=on  InputSameDT=on
  Switch1 : Switch  Orientation=left  SaturateOnIntegerOverflow=on  InputSameDT=on
  inv. : Fcn  Orientation=left  Expr=1/u
  neg : Gain  Orientation=left  Gain=-1  SaturateOnIntegerOverflow=on
  neg1 : Gain  Orientation=left  Gain=-1  SaturateOnIntegerOverflow=on
  out_1 : Outport  Orientation=left  InitialOutput=0
  wires:
  Switch/1 -> out_1/1
  neg/1 -> Switch/2
  Constant/1 -> Switch/1
  inv./1 -> Switch/3
  Switch1/1 -> inv./1
  neg1/1 -> Switch1/2
  Constant1/1 -> Switch1/1
  in_1/1 -> neg/1, neg1/1, Switch1/3

== system SEWSYS_Combined/Sewage plant/Screen/Separation/3-6 ==
  in_1 : Inport  Orientation=down  Port=1  LatchInput=off
  "in_2 " : Inport  Orientation=down  Port=2  LatchInput=off
  Ground : Ground  Orientation=down
  Mux : Mux  Orientation=down
  N-tot : MATLABFcn  Orientation=down  MATLABFcn=(u(1)-u(2)-u(3))*SSred_screen  OutputDimensions=1
  NH4 : Product  Orientation=down  SaturateOnIntegerOverflow=on  InputSameDT=on
  "NH4 " : Fcn  Orientation=down  Expr=u(2)
  NH5 : Product  Orientation=down  SaturateOnIntegerOverflow=on  InputSameDT=on
  NO3 : Fcn  Orientation=down  Expr=u(3)
  Sum : Sum  Orientation=down  Inputs=+++  SaturateOnIntegerOverflow=on  InputSameDT=on
  out_1 : Outport  Orientation=down  InitialOutput=0
  wires:
  NH4/1 -> Mux/2, Sum/2
  in_1/1 -> NH5/1, NH4/1
  Mux/1 -> out_1/1
  N-tot/1 -> Sum/1
  Sum/1 -> Mux/1
  "NH4 "/1 -> NH4/2
  NO3/1 -> NH5/2
  "in_2 "/1 -> NO3/1, "NH4 "/1, N-tot/1
  NH5/1 -> Sum/3, Mux/3
  Ground/1 -> Mux/4

== system SEWSYS_Combined/Sewage plant/Screen/Separation/if u>0 then 1/u else 0 ==
  note: if u<=0, 0, else 1/u, end
  in_1 : Inport  Orientation=left  Port=1  LatchInput=off
  Constant : Constant  Orientation=left  Value=0
  Constant1 : Constant  Orientation=left
  Switch : Switch  Orientation=left  SaturateOnIntegerOverflow=on  InputSameDT=on
  Switch1 : Switch  Orientation=left  SaturateOnIntegerOverflow=on  InputSameDT=on
  inv. : Fcn  Orientation=left  Expr=1/u
  neg : Gain  Orientation=left  Gain=-1  SaturateOnIntegerOverflow=on
  neg1 : Gain  Orientation=left  Gain=-1  SaturateOnIntegerOverflow=on
  out_1 : Outport  Orientation=left  InitialOutput=0
  wires:
  Constant/1 -> Switch/1
  neg/1 -> Switch/2
  Switch/1 -> out_1/1
  inv./1 -> Switch/3
  Switch1/1 -> inv./1
  neg1/1 -> Switch1/2
  Constant1/1 -> Switch1/1
  in_1/1 -> neg/1, neg1/1, Switch1/3
